simulink model "WaveletTraj"  (Simulink 10.1)
settings: Solver=FixedStepDiscrete  StartTime=0.0  StopTime=inf  FixedStep=Ts  RelTol=1e-3
PreLoadFcn:
  | load param
undefined symbols (not defined in the file or in its folder): c_maxsz, DiscIntNeverNeededParam, Dphival_fi, f, interp_gain, interp_uplim, phival_fi, Ts, tval_fi, w
libraries: simulink x36, dspsigops x24, dspindex x16, dspswit3 x12, simulink_extras x8
(part 2 of 4)

== system WaveletTraj/Wavelet Trajectory/TrajGen1/Input Latching ==
  trigger : Inport
  abort : Inport  Port=2
  mode : Inport  Port=3
  int_mode : Inport  Port=4
  Res : Inport  Port=5
  x0 : Inport  Port=6
  xf : Inport  Port=7
  T : Inport  Port=8
  c : Inport  Port=9
  Edge Detector : dspswit3/Edge Detector  SystemSampleTime=-1
      settings: SourceProductBaseCode=DS
  Edge Detector1 : dspswit3/Edge Detector  SystemSampleTime=-1
      settings: SourceProductBaseCode=DS
  Sample and Hold : Subsystem  TreatAsAtomicUnit=on  mask(Sample and Hold){trig=Rising edge, initCond=0, latchinput=off}
      mask prompts: trig "Trigger type:"; initCond "Initial condition:"; latchinput "Latch (buffer) input"
      mask help: Sample and hold the input signal. If Latch (buffer) input is selected, then this block produces the value of the input from the previous time step.
      mask init:
      | switch trig
      | case 1, s='rising';
      | case 2, s='falling';
      | case 3, s='either';
      | end
      | set_param([gcb '/Trigger'],'triggertype',s);
      | if (latchinput == 1)
      | 	set_param([gcb '/In'],'latchinput','on');
      | 	set_param([gcb '/mode'],'latchinput','on');
      | else
      | 	set_param([gcb '/In'],'latchinput','off');
      | 	set_param([gcb '/mode'],'latchinput','off');
      | end
      mask Help: eval('blocksethelp');
      mask TypeOptions trig: Rising edge | Falling edge | Either edge
      mask Display: disp('S/H')
  Sample and Hold1 : dspsigops/Sample and Hold  SystemSampleTime=-1  trig=Rising edge  initCond=0  latchinput=off
  Sample and Hold2 : Subsystem  TreatAsAtomicUnit=on  mask(Sample and Hold){trig=Rising edge, initCond=0, latchinput=off}
      mask prompts: trig "Trigger type:"; initCond "Initial condition:"; latchinput "Latch (buffer) input"
      mask help: Sample and hold the input signal. If Latch (buffer) input is selected, then this block produces the value of the input from the previous time step.
      mask init:
      | switch trig
      | case 1, s='rising';
      | case 2, s='falling';
      | case 3, s='either';
      | end
      | set_param([gcb '/Trigger'],'triggertype',s);
      | if (latchinput == 1)
      | 	set_param([gcb '/In'],'latchinput','on');
      | else
      | 	set_param([gcb '/In'],'latchinput','off');
      | end
      mask Help: eval('blocksethelp');
      mask TypeOptions trig: Rising edge | Falling edge | Either edge
      mask Display: disp('S/H')
  Sample and Hold3 : dspsigops/Sample and Hold  SystemSampleTime=-1  trig=Rising edge  initCond=0  latchinput=off
  Sample and Hold4 : Subsystem  TreatAsAtomicUnit=on  mask(Sample and Hold){trig=Rising edge, initCond=0, latchinput=off}
      mask prompts: trig "Trigger type:"; initCond "Initial condition:"; latchinput "Latch (buffer) input"
      mask help: Sample and hold the input signal. If Latch (buffer) input is selected, then this block produces the value of the input from the previous time step.
      mask init: same as WaveletTraj/Wavelet Trajectory/TrajGen1/Input Latching/Sample and Hold
      mask Help: eval('blocksethelp');
      mask TypeOptions trig: Rising edge | Falling edge | Either edge
      mask Display: disp('S/H')
  Sample and Hold5 : Subsystem  TreatAsAtomicUnit=on  mask(Sample and Hold){trig=Rising edge, initCond=0, latchinput=off}
      mask prompts: trig "Trigger type:"; initCond "Initial condition:"; latchinput "Latch (buffer) input"
      mask help: Sample and hold the input signal. If Latch (buffer) input is selected, then this block produces the value of the input from the previous time step.
      mask init:
      | switch trig
      | case 1, s='rising';
      | case 2, s='falling';
      | case 3, s='either';
      | end
      | set_param([gcb '/Trigger'],'triggertype',s);
      | if (latchinput == 1)
      | 	set_param([gcb '/mode'],'latchinput','on');
      | 	set_param([gcb '/x0'],'latchinput','on');
      | 	set_param([gcb '/xf'],'latchinput','on');
      | else
      | 	set_param([gcb '/mode'],'latchinput','off');
      | 	set_param([gcb '/x0'],'latchinput','off');
      | 	set_param([gcb '/xf'],'latchinput','off');
      | end
      mask Help: eval('blocksethelp');
      mask TypeOptions trig: Rising edge | Falling edge | Either edge
      mask Display: disp('S/H')
  Sample and Hold6 : dspsigops/Sample and Hold  SystemSampleTime=-1  trig=Rising edge  initCond=0  latchinput=off
  Saturation : Saturate  UpperLimit=2  LowerLimit=0  OutDataTypeStr=uint8  RndMeth=Nearest
  trigger_trg : Outport
  abort_trg : Outport  Port=2
  mode_lt : Outport  Port=3
  int_mode_lt : Outport  Port=4
  Res_lt : Outport  Port=5
  N_lt : Outport  Port=6
  x0_lt : Outport  Port=7
  mul_lt : Outport  Port=8
  T1 : Outport  Port=9
  c_lt : Outport  Port=10
  wires:
  Sample and Hold4/1(" ") -> c_lt/1
  Sample and Hold2/1(" ") -> T1/1
  T/1 -> Sample and Hold2/1(In)
  Sample and Hold1/1 -> x0_lt/1
  x0/1 -> Sample and Hold1/1, Sample and Hold5/2(x0)
  Sample and Hold/2(" 1") -> N_lt/1
  Res/1 -> Sample and Hold/2(In)
  Sample and Hold/1(" ") -> Res_lt/1
  Edge Detector/1 -> trigger_trg/1
  trigger/1 -> Edge Detector/1, Sample and Hold3/Trigger, Sample and Hold1/Trigger, Sample and Hold5/Trigger, Sample and Hold2/Trigger, Sample and Hold4/Trigger, Sample and Hold/Trigger, Sample and Hold6/Trigger
  mode/1 -> Saturation/1
  xf/1 -> Sample and Hold5/3(xf)
  Sample and Hold5/1(" ") -> mul_lt/1
  c/1 -> Sample and Hold4/2(In)
  abort/1 -> Edge Detector1/1
  Edge Detector1/1 -> abort_trg/1
  Sample and Hold3/1 -> mode_lt/1
  Sample and Hold6/1 -> int_mode_lt/1
  int_mode/1 -> Sample and Hold6/1
  Saturation/1 -> Sample and Hold4/1(mode), Sample and Hold5/1(mode), Sample and Hold/1(mode), Sample and Hold3/1

== system WaveletTraj/Wavelet Trajectory/TrajGen2/Compute Join Coeffs ==
  x_z1 : Inport
  tau_z1 : Inport  Port=2
  Res_z1 : Inport  Port=3
  c_z1 : Inport  Port=4
  N_z1 : Inport  Port=5
  mul_z1 : Inport  Port=6
  Res : Inport  Port=7
  c : Inport  Port=8
  N : Inport  Port=9
  mul : Inport  Port=10
  x0 : Inport  Port=11
  Trigger : TriggerPort  VariantControl=(inherit)  StatesWhenEnabling=reset
  Abs : Abs  RndMeth=Nearest  SaturateOnIntegerOverflow=on
  Constant : Constant  Value=0  OutDataTypeStr=fixdt(1,w,f)
  Derivative1 in tau : Subsystem  TreatAsAtomicUnit=on  RTWFcnName=Trajectory_Derivative
      settings: RTWFcnNameOpts=User specified
  Derivative2 in 0 : Subsystem  TreatAsAtomicUnit=on  RTWFcnName=Trajectory_Derivative
      settings: RTWFcnNameOpts=User specified
  Derivative2 in tau1 : Subsystem  TreatAsAtomicUnit=on  RTWFcnName=Trajectory_Derivative
      settings: RTWFcnNameOpts=User specified
  Find Coeffs : Subsystem  TreatAsAtomicUnit=on  RTWFcnName=Trajectory_FindCoeffs
      settings: RTWFcnNameOpts=User specified
  Gain : Gain  Gain=interp_gain  ParamDataTypeStr=fixdt(1,w,f)  RndMeth=Nearest  SaturateOnIntegerOverflow=on  OutDataTypeStr=Inherit: Same as input
  Position2 in tau1 : Subsystem  TreatAsAtomicUnit=on  RTWFcnName=Trajectory_Position
      settings: RTWFcnNameOpts=User specified
  Product{,1..3} (4 alike) : Product  OutDataTypeStr=fixdt(1,w,f)  RndMeth=Nearest  SaturateOnIntegerOverflow=on
  Saturation1 : Saturate  UpperLimit=interp_uplim  LowerLimit=0  OutDataTypeStr=fixdt(1,w,f)  RndMeth=Nearest
  Sum1 : Sum  Inputs=++|  OutDataTypeStr=fixdt(1,w,f)  RndMeth=Nearest  SaturateOnIntegerOverflow=on
  Sum2 : Sum  Inputs=|+-  OutDataTypeStr=fixdt(1,w,f)  RndMeth=Nearest  SaturateOnIntegerOverflow=on
  tau1 : Outport
  DET_OK : Outport  Port=2
  Coeffs : Outport  Port=3
  wires:
  mul/1 -> Product3/1, Product/1, Product2/1
  Position2 in tau1/1(out) -> Product/2
  Product3/1 -> [Dout2]
  Derivative2 in tau1/1(out) -> Product3/2
  Product2/1 -> Sum2/2
  Derivative2 in 0/1(out) -> Product2/2
  mul_z1/1 -> Product1/1
  Product1/1 -> [Dout1], Sum2/1
  Derivative1 in tau/1(out) -> Product1/2
  Product/1 -> Sum1/2
  Res/1 -> Position2 in tau1/1(Res), Derivative2 in tau1/1(Res), Derivative2 in 0/1(Res)
  Constant/1 -> Derivative2 in 0/2(tau)
  c/1 -> Position2 in tau1/3(c), Derivative2 in tau1/3(c), Derivative2 in 0/3(c)
  N/1 -> Position2 in tau1/4(N), Derivative2 in tau1/4(N), Derivative2 in 0/4(N)
  Sum2/1 -> Abs/1
  Abs/1 -> Gain/1
  Gain/1 -> Saturation1/1
  [tau1] -> Position2 in tau1/2(tau), Derivative2 in tau1/2(tau)
  x_z1/1 -> [out1]
  [tau1] -> Find Coeffs/1(tau1)
  [out1] -> Find Coeffs/2(out1)
  [Dout1] -> Find Coeffs/3(Dout1)
  [out2] -> Find Coeffs/4(out2)
  [Dout2] -> Find Coeffs/5(Dout2)
  Find Coeffs/2(Coeffs) -> Coeffs/1
  Saturation1/1 -> tau1/1, [tau1]
  Sum1/1 -> [out2]
  x0/1 -> Sum1/1
  c_z1/1 -> Derivative1 in tau/3(c)
  tau_z1/1 -> Derivative1 in tau/2(tau)
  Find Coeffs/1(DET_OK) -> DET_OK/1
  Res_z1/1 -> Derivative1 in tau/1(Res)
  N_z1/1 -> Derivative1 in tau/4(N)

== system WaveletTraj/Wavelet Trajectory/TrajGen2/Compute Join Output ==
  Coeffs : Inport
  tau : Inport  Port=2
  tau1 : Inport  Port=3
  x : Inport  Port=4
  Enable : EnablePort
  CalcPoly : Subsystem
  CalcRho : Subsystem
  Product : Product  OutDataTypeStr=fixdt(1,w,f)  RndMeth=Nearest  SaturateOnIntegerOverflow=on
  Product1 : Product  OutDataTypeStr=fixdt(1,w,f)  RndMeth=Nearest  SaturateOnIntegerOverflow=on
  Sum2 : Sum  Inputs=|++  OutDataTypeStr=fixdt(1,w,f)  RndMeth=Nearest  SaturateOnIntegerOverflow=on
  x_join : Outport
  wires:
  tau/1 -> CalcPoly/1(tau), CalcRho/1(tau)
  Coeffs/1 -> CalcPoly/2(Coeffs)
  tau1/1 -> CalcRho/2(tau1)
  CalcPoly/1(out_poly3) -> Product/1
  CalcRho/1(Rho1) -> Product/2
  Product/1 -> Sum2/1
  Product1/1 -> Sum2/2
  Sum2/1 -> x_join/1
  CalcRho/2(Rho2) -> Product1/1
  x/1 -> Product1/2

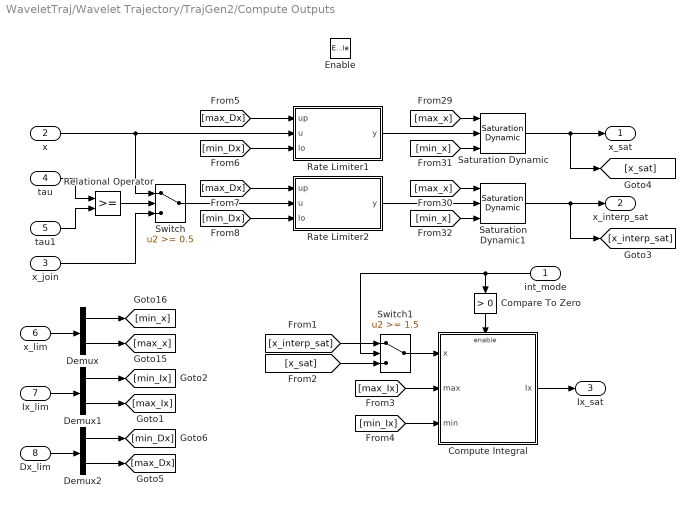
== system WaveletTraj/Wavelet Trajectory/TrajGen2/Compute Outputs ==
  int_mode : Inport
  x : Inport  Port=2
  x_join : Inport  Port=3
  tau : Inport  Port=4
  tau1 : Inport  Port=5
  x_lim : Inport  Port=6
  Ix_lim : Inport  Port=7
  Dx_lim : Inport  Port=8
  Enable : EnablePort
  Compare To Zero : simulink/Logic and Bit Operations/Compare To Zero  SystemSampleTime=-1  relop=>  LogicOutDataTypeMode=boolean  ZeroCross=off
  Compute Integral : Subsystem  TreatAsAtomicUnit=on  RTWFcnName=Trajectory_ComputeIntegral
      settings: RTWFcnNameOpts=User specified
  Demux : Demux  Outputs=2
  Demux1 : Demux  Outputs=2
  Demux2 : Demux  Outputs=2
  Rate Limiter1 : Subsystem  TreatAsAtomicUnit=on  RTWFcnName=Trajectory_RateLimiter
      settings: RTWFcnNameOpts=User specified
      mask Display:
      | disp('Rate\nLimiter');
      | port_label('input',1,'up');
      | port_label('input',2,'u');
      | port_label('input',3,'lo');
      | port_label('output',1,'y');
  Rate Limiter2 : Subsystem  TreatAsAtomicUnit=on  RTWFcnName=Trajectory_RateLimiter
      settings: RTWFcnNameOpts=User specified
      mask Display:
      | disp('Rate\nLimiter');
      | port_label('input',1,'up');
      | port_label('input',2,'u');
      | port_label('input',3,'lo');
      | port_label('output',1,'y');
  Relational Operator : RelationalOperator  OutDataTypeStr=boolean  RndMeth=Nearest
  Saturation Dynamic : simulink/Discontinuities/Saturation Dynamic  SystemSampleTime=-1  OutMin=[]  OutMax=[]  OutDataTypeStr=fixdt(1,w,f)  OutputDataTypeScalingMode=Specify via dialog  OutDataType=fixdt(1,w,f)  OutScaling=[]  RndMeth=Nearest  DoSatur=on
  Saturation Dynamic1 : simulink/Discontinuities/Saturation Dynamic  SystemSampleTime=-1  OutMin=[]  OutMax=[]  OutDataTypeStr=fixdt(1,w,f)  OutputDataTypeScalingMode=Specify via dialog  OutDataType=fixdt(1,w,f)  OutScaling=[]  RndMeth=Nearest  DoSatur=on
  Switch : Switch  Threshold=0.5  OutDataTypeStr=fixdt(1,w,f)  RndMeth=Nearest  SaturateOnIntegerOverflow=on
  Switch1 : Switch  Threshold=1.5  OutDataTypeStr=fixdt(1,w,f)  RndMeth=Nearest  SaturateOnIntegerOverflow=on
  x_sat : Outport
  x_interp_sat : Outport  Port=2
  Ix_sat : Outport  Port=3
  wires:
  [max_Dx] -> Rate Limiter2/1(up)
  [min_Dx] -> Rate Limiter2/3(lo)
  [min_Dx] -> Rate Limiter1/3(lo)
  [max_Dx] -> Rate Limiter1/1(up)
  Switch/1 -> Rate Limiter2/2(u)
  Rate Limiter2/1(y) -> Saturation Dynamic1/2
  Rate Limiter1/1(y) -> Saturation Dynamic/2
  Dx_lim/1 -> Demux2/1
  Demux2/2 -> [max_Dx]
  Demux2/1 -> [min_Dx]
  Compare To Zero/1 -> Compute Integral/Enable
  int_mode/1 -> Switch1/2, Compare To Zero/1
  Switch1/1 -> Compute Integral/1(x)
  [x_sat] -> Switch1/3
  [x_interp_sat] -> Switch1/1
  Ix_lim/1 -> Demux1/1
  x_lim/1 -> Demux/1
  Compute Integral/1(Ix) -> Ix_sat/1
  [min_Ix] -> Compute Integral/3(min)
  [max_Ix] -> Compute Integral/2(max)
  Demux1/2 -> [max_Ix]
  Demux1/1 -> [min_Ix]
  Demux/2 -> [max_x]
  Demux/1 -> [min_x]
  x_join/1 -> Switch/3
  tau1/1 -> Relational Operator/2
  Saturation Dynamic1/1 -> [x_interp_sat], x_interp_sat/1
  tau/1 -> Relational Operator/1
  Saturation Dynamic/1 -> [x_sat], x_sat/1
  Relational Operator/1 -> Switch/2
  [max_x] -> Saturation Dynamic/1
  [max_x] -> Saturation Dynamic1/1
  [min_x] -> Saturation Dynamic/3
  [min_x] -> Saturation Dynamic1/3
  x/1 -> Rate Limiter1/2(u), Switch/1

== system WaveletTraj/Wavelet Trajectory/TrajGen2/Compute Position ==
  Res : Inport  PortDimensions=1
  tau : Inport  Port=2  PortDimensions=1
  c : Inport  Port=3  PortDimensions=c_maxsz
  N : Inport  Port=4  PortDimensions=1
  mul : Inport  Port=5  PortDimensions=1
  x0 : Inport  Port=6  PortDimensions=1
  Enable : EnablePort
  Position : Subsystem  TreatAsAtomicUnit=on  RTWFcnName=Trajectory_Position
      settings: RTWFcnNameOpts=User specified
  Product : Product  OutDataTypeStr=fixdt(1,w,f)  RndMeth=Nearest  SaturateOnIntegerOverflow=on
  Sum1 : Sum  Inputs=|++  OutDataTypeStr=fixdt(1,w,f)  RndMeth=Nearest  SaturateOnIntegerOverflow=on
  out : Outport  PortDimensions=1
  wires:
  mul/1 -> Product/2
  Product/1 -> Sum1/1
  Position/1(out) -> Product/1
  Res/1 -> Position/1(Res)
  tau/1 -> Position/2(tau)
  c/1 -> Position/3(c)
  N/1 -> Position/4(N)
  Sum1/1 -> out/1
  x0/1 -> Sum1/2

== system WaveletTraj/Wavelet Trajectory/TrajGen2/Input Latching ==
  trigger : Inport
  abort : Inport  Port=2
  mode : Inport  Port=3
  int_mode : Inport  Port=4
  Res : Inport  Port=5
  x0 : Inport  Port=6
  xf : Inport  Port=7
  T : Inport  Port=8
  c : Inport  Port=9
  Edge Detector : dspswit3/Edge Detector  SystemSampleTime=-1
      settings: SourceProductBaseCode=DS
  Edge Detector1 : dspswit3/Edge Detector  SystemSampleTime=-1
      settings: SourceProductBaseCode=DS
  Sample and Hold : Subsystem  TreatAsAtomicUnit=on  mask(Sample and Hold){trig=Rising edge, initCond=0, latchinput=off}
      mask prompts: trig "Trigger type:"; initCond "Initial condition:"; latchinput "Latch (buffer) input"
      mask help: Sample and hold the input signal. If Latch (buffer) input is selected, then this block produces the value of the input from the previous time step.
      mask init: same as WaveletTraj/Wavelet Trajectory/TrajGen1/Input Latching/Sample and Hold
      mask Help: eval('blocksethelp');
      mask TypeOptions trig: Rising edge | Falling edge | Either edge
      mask Display: disp('S/H')
  Sample and Hold1 : dspsigops/Sample and Hold  SystemSampleTime=-1  trig=Rising edge  initCond=0  latchinput=off
  Sample and Hold2 : Subsystem  TreatAsAtomicUnit=on  mask(Sample and Hold){trig=Rising edge, initCond=0, latchinput=off}
      mask prompts: trig "Trigger type:"; initCond "Initial condition:"; latchinput "Latch (buffer) input"
      mask help: Sample and hold the input signal. If Latch (buffer) input is selected, then this block produces the value of the input from the previous time step.
      mask init: same as WaveletTraj/Wavelet Trajectory/TrajGen1/Input Latching/Sample and Hold2
      mask Help: eval('blocksethelp');
      mask TypeOptions trig: Rising edge | Falling edge | Either edge
      mask Display: disp('S/H')
  Sample and Hold3 : dspsigops/Sample and Hold  SystemSampleTime=-1  trig=Rising edge  initCond=0  latchinput=off
  Sample and Hold4 : Subsystem  TreatAsAtomicUnit=on  mask(Sample and Hold){trig=Rising edge, initCond=0, latchinput=off}
      mask prompts: trig "Trigger type:"; initCond "Initial condition:"; latchinput "Latch (buffer) input"
      mask help: Sample and hold the input signal. If Latch (buffer) input is selected, then this block produces the value of the input from the previous time step.
      mask init: same as WaveletTraj/Wavelet Trajectory/TrajGen1/Input Latching/Sample and Hold
      mask Help: eval('blocksethelp');
      mask TypeOptions trig: Rising edge | Falling edge | Either edge
      mask Display: disp('S/H')
  Sample and Hold5 : Subsystem  TreatAsAtomicUnit=on  mask(Sample and Hold){trig=Rising edge, initCond=0, latchinput=off}
      mask prompts: trig "Trigger type:"; initCond "Initial condition:"; latchinput "Latch (buffer) input"
      mask help: Sample and hold the input signal. If Latch (buffer) input is selected, then this block produces the value of the input from the previous time step.
      mask init: same as WaveletTraj/Wavelet Trajectory/TrajGen1/Input Latching/Sample and Hold5
      mask Help: eval('blocksethelp');
      mask TypeOptions trig: Rising edge | Falling edge | Either edge
      mask Display: disp('S/H')
  Sample and Hold6 : dspsigops/Sample and Hold  SystemSampleTime=-1  trig=Rising edge  initCond=0  latchinput=off
  Saturation : Saturate  UpperLimit=2  LowerLimit=0  OutDataTypeStr=uint8  RndMeth=Nearest
  trigger_trg : Outport
  abort_trg : Outport  Port=2
  mode_lt : Outport  Port=3
  int_mode_lt : Outport  Port=4
  Res_lt : Outport  Port=5
  N_lt : Outport  Port=6
  x0_lt : Outport  Port=7
  mul_lt : Outport  Port=8
  T1 : Outport  Port=9
  c_lt : Outport  Port=10
  wires:
  Saturation/1 -> Sample and Hold3/1, Sample and Hold/1(mode), Sample and Hold5/1(mode), Sample and Hold4/1(mode)
  int_mode/1 -> Sample and Hold6/1
  Sample and Hold6/1 -> int_mode_lt/1
  Sample and Hold3/1 -> mode_lt/1
  Edge Detector1/1 -> abort_trg/1
  abort/1 -> Edge Detector1/1
  c/1 -> Sample and Hold4/2(In)
  Sample and Hold5/1(" ") -> mul_lt/1
  xf/1 -> Sample and Hold5/3(xf)
  mode/1 -> Saturation/1
  trigger/1 -> Sample and Hold6/Trigger, Sample and Hold/Trigger, Sample and Hold4/Trigger, Sample and Hold2/Trigger, Sample and Hold5/Trigger, Sample and Hold1/Trigger, Sample and Hold3/Trigger, Edge Detector/1
  Edge Detector/1 -> trigger_trg/1
  Sample and Hold/1(" ") -> Res_lt/1
  Res/1 -> Sample and Hold/2(In)
  Sample and Hold/2(" 1") -> N_lt/1
  x0/1 -> Sample and Hold5/2(x0), Sample and Hold1/1
  Sample and Hold1/1 -> x0_lt/1
  T/1 -> Sample and Hold2/1(In)
  Sample and Hold2/1(" ") -> T1/1
  Sample and Hold4/1(" ") -> c_lt/1

== system WaveletTraj/Wavelet Trajectory/TrajGen3/Compute Join Coeffs ==
  x_z1 : Inport
  tau_z1 : Inport  Port=2
  Res_z1 : Inport  Port=3
  c_z1 : Inport  Port=4
  N_z1 : Inport  Port=5
  mul_z1 : Inport  Port=6
  Res : Inport  Port=7
  c : Inport  Port=8
  N : Inport  Port=9
  mul : Inport  Port=10
  x0 : Inport  Port=11
  Trigger : TriggerPort  VariantControl=(inherit)  StatesWhenEnabling=reset
  Abs : Abs  RndMeth=Nearest  SaturateOnIntegerOverflow=on
  Constant : Constant  Value=0  OutDataTypeStr=fixdt(1,w,f)
  Derivative1 in tau : Subsystem  TreatAsAtomicUnit=on  RTWFcnName=Trajectory_Derivative
      settings: RTWFcnNameOpts=User specified
  Derivative2 in 0 : Subsystem  TreatAsAtomicUnit=on  RTWFcnName=Trajectory_Derivative
      settings: RTWFcnNameOpts=User specified
  Derivative2 in tau1 : Subsystem  TreatAsAtomicUnit=on  RTWFcnName=Trajectory_Derivative
      settings: RTWFcnNameOpts=User specified
  Find Coeffs : Subsystem  TreatAsAtomicUnit=on  RTWFcnName=Trajectory_FindCoeffs
      settings: RTWFcnNameOpts=User specified
  Gain : Gain  Gain=interp_gain  ParamDataTypeStr=fixdt(1,w,f)  RndMeth=Nearest  SaturateOnIntegerOverflow=on  OutDataTypeStr=Inherit: Same as input
  Position2 in tau1 : Subsystem  TreatAsAtomicUnit=on  RTWFcnName=Trajectory_Position
      settings: RTWFcnNameOpts=User specified
  Product{,1..3} (4 alike) : Product  OutDataTypeStr=fixdt(1,w,f)  RndMeth=Nearest  SaturateOnIntegerOverflow=on
  Saturation1 : Saturate  UpperLimit=interp_uplim  LowerLimit=0  OutDataTypeStr=fixdt(1,w,f)  RndMeth=Nearest
  Sum1 : Sum  Inputs=++|  OutDataTypeStr=fixdt(1,w,f)  RndMeth=Nearest  SaturateOnIntegerOverflow=on
  Sum2 : Sum  Inputs=|+-  OutDataTypeStr=fixdt(1,w,f)  RndMeth=Nearest  SaturateOnIntegerOverflow=on
  tau1 : Outport
  DET_OK : Outport  Port=2
  Coeffs : Outport  Port=3
  wires:
  N_z1/1 -> Derivative1 in tau/4(N)
  Res_z1/1 -> Derivative1 in tau/1(Res)
  Find Coeffs/1(DET_OK) -> DET_OK/1
  tau_z1/1 -> Derivative1 in tau/2(tau)
  c_z1/1 -> Derivative1 in tau/3(c)
  x0/1 -> Sum1/1
  Sum1/1 -> [out2]
  Saturation1/1 -> [tau1], tau1/1
  Find Coeffs/2(Coeffs) -> Coeffs/1
  [Dout2] -> Find Coeffs/5(Dout2)
  [out2] -> Find Coeffs/4(out2)
  [Dout1] -> Find Coeffs/3(Dout1)
  [out1] -> Find Coeffs/2(out1)
  [tau1] -> Find Coeffs/1(tau1)
  x_z1/1 -> [out1]
  [tau1] -> Derivative2 in tau1/2(tau), Position2 in tau1/2(tau)
  Gain/1 -> Saturation1/1
  Abs/1 -> Gain/1
  Sum2/1 -> Abs/1
  N/1 -> Derivative2 in 0/4(N), Derivative2 in tau1/4(N), Position2 in tau1/4(N)
  c/1 -> Derivative2 in 0/3(c), Derivative2 in tau1/3(c), Position2 in tau1/3(c)
  Constant/1 -> Derivative2 in 0/2(tau)
  Res/1 -> Derivative2 in 0/1(Res), Derivative2 in tau1/1(Res), Position2 in tau1/1(Res)
  Product/1 -> Sum1/2
  Derivative1 in tau/1(out) -> Product1/2
  Product1/1 -> Sum2/1, [Dout1]
  mul_z1/1 -> Product1/1
  Derivative2 in 0/1(out) -> Product2/2
  Product2/1 -> Sum2/2
  Derivative2 in tau1/1(out) -> Product3/2
  Product3/1 -> [Dout2]
  Position2 in tau1/1(out) -> Product/2
  mul/1 -> Product2/1, Product/1, Product3/1

== system WaveletTraj/Wavelet Trajectory/TrajGen3/Compute Join Output ==
  Coeffs : Inport
  tau : Inport  Port=2
  tau1 : Inport  Port=3
  x : Inport  Port=4
  Enable : EnablePort
  CalcPoly : Subsystem
  CalcRho : Subsystem
  Product : Product  OutDataTypeStr=fixdt(1,w,f)  RndMeth=Nearest  SaturateOnIntegerOverflow=on
  Product1 : Product  OutDataTypeStr=fixdt(1,w,f)  RndMeth=Nearest  SaturateOnIntegerOverflow=on
  Sum2 : Sum  Inputs=|++  OutDataTypeStr=fixdt(1,w,f)  RndMeth=Nearest  SaturateOnIntegerOverflow=on
  x_join : Outport
  wires:
  x/1 -> Product1/2
  CalcRho/2(Rho2) -> Product1/1
  Sum2/1 -> x_join/1
  Product1/1 -> Sum2/2
  Product/1 -> Sum2/1
  CalcRho/1(Rho1) -> Product/2
  CalcPoly/1(out_poly3) -> Product/1
  tau1/1 -> CalcRho/2(tau1)
  Coeffs/1 -> CalcPoly/2(Coeffs)
  tau/1 -> CalcRho/1(tau), CalcPoly/1(tau)

== system WaveletTraj/Wavelet Trajectory/TrajGen3/Compute Outputs ==
  int_mode : Inport
  x : Inport  Port=2
  x_join : Inport  Port=3
  tau : Inport  Port=4
  tau1 : Inport  Port=5
  x_lim : Inport  Port=6
  Ix_lim : Inport  Port=7
  Dx_lim : Inport  Port=8
  Enable : EnablePort
  Compare To Zero : simulink/Logic and Bit Operations/Compare To Zero  SystemSampleTime=-1  relop=>  LogicOutDataTypeMode=boolean  ZeroCross=off
  Compute Integral : Subsystem  TreatAsAtomicUnit=on  RTWFcnName=Trajectory_ComputeIntegral
      settings: RTWFcnNameOpts=User specified
  Demux : Demux  Outputs=2
  Demux1 : Demux  Outputs=2
  Demux2 : Demux  Outputs=2
  Rate Limiter1 : Subsystem  TreatAsAtomicUnit=on  RTWFcnName=Trajectory_RateLimiter
      settings: RTWFcnNameOpts=User specified
      mask Display:
      | disp('Rate\nLimiter');
      | port_label('input',1,'up');
      | port_label('input',2,'u');
      | port_label('input',3,'lo');
      | port_label('output',1,'y');
  Rate Limiter2 : Subsystem  TreatAsAtomicUnit=on  RTWFcnName=Trajectory_RateLimiter
      settings: RTWFcnNameOpts=User specified
      mask Display:
      | disp('Rate\nLimiter');
      | port_label('input',1,'up');
      | port_label('input',2,'u');
      | port_label('input',3,'lo');
      | port_label('output',1,'y');
  Relational Operator : RelationalOperator  OutDataTypeStr=boolean  RndMeth=Nearest
  Saturation Dynamic : simulink/Discontinuities/Saturation Dynamic  SystemSampleTime=-1  OutMin=[]  OutMax=[]  OutDataTypeStr=fixdt(1,w,f)  OutputDataTypeScalingMode=Specify via dialog  OutDataType=fixdt(1,w,f)  OutScaling=[]  RndMeth=Nearest  DoSatur=on
  Saturation Dynamic1 : simulink/Discontinuities/Saturation Dynamic  SystemSampleTime=-1  OutMin=[]  OutMax=[]  OutDataTypeStr=fixdt(1,w,f)  OutputDataTypeScalingMode=Specify via dialog  OutDataType=fixdt(1,w,f)  OutScaling=[]  RndMeth=Nearest  DoSatur=on
  Switch : Switch  Threshold=0.5  OutDataTypeStr=fixdt(1,w,f)  RndMeth=Nearest  SaturateOnIntegerOverflow=on
  Switch1 : Switch  Threshold=1.5  OutDataTypeStr=fixdt(1,w,f)  RndMeth=Nearest  SaturateOnIntegerOverflow=on
  x_sat : Outport
  x_interp_sat : Outport  Port=2
  Ix_sat : Outport  Port=3
  wires:
  x/1 -> Switch/1, Rate Limiter1/2(u)
  [min_x] -> Saturation Dynamic1/3
  [min_x] -> Saturation Dynamic/3
  [max_x] -> Saturation Dynamic1/1
  [max_x] -> Saturation Dynamic/1
  Relational Operator/1 -> Switch/2
  Saturation Dynamic/1 -> x_sat/1, [x_sat]
  tau/1 -> Relational Operator/1
  Saturation Dynamic1/1 -> x_interp_sat/1, [x_interp_sat]
  tau1/1 -> Relational Operator/2
  x_join/1 -> Switch/3
  Demux/1 -> [min_x]
  Demux/2 -> [max_x]
  Demux1/1 -> [min_Ix]
  Demux1/2 -> [max_Ix]
  [max_Ix] -> Compute Integral/2(max)
  [min_Ix] -> Compute Integral/3(min)
  Compute Integral/1(Ix) -> Ix_sat/1
  x_lim/1 -> Demux/1
  Ix_lim/1 -> Demux1/1
  [x_interp_sat] -> Switch1/1
  [x_sat] -> Switch1/3
  Switch1/1 -> Compute Integral/1(x)
  int_mode/1 -> Compare To Zero/1, Switch1/2
  Compare To Zero/1 -> Compute Integral/Enable
  Demux2/1 -> [min_Dx]
  Demux2/2 -> [max_Dx]
  Dx_lim/1 -> Demux2/1
  Rate Limiter1/1(y) -> Saturation Dynamic/2
  Rate Limiter2/1(y) -> Saturation Dynamic1/2
  Switch/1 -> Rate Limiter2/2(u)
  [max_Dx] -> Rate Limiter1/1(up)
  [min_Dx] -> Rate Limiter1/3(lo)
  [min_Dx] -> Rate Limiter2/3(lo)
  [max_Dx] -> Rate Limiter2/1(up)

== system WaveletTraj/Wavelet Trajectory/TrajGen3/Compute Position ==
  Res : Inport  PortDimensions=1
  tau : Inport  Port=2  PortDimensions=1
  c : Inport  Port=3  PortDimensions=c_maxsz
  N : Inport  Port=4  PortDimensions=1
  mul : Inport  Port=5  PortDimensions=1
  x0 : Inport  Port=6  PortDimensions=1
  Enable : EnablePort
  Position : Subsystem  TreatAsAtomicUnit=on  RTWFcnName=Trajectory_Position
      settings: RTWFcnNameOpts=User specified
  Product : Product  OutDataTypeStr=fixdt(1,w,f)  RndMeth=Nearest  SaturateOnIntegerOverflow=on
  Sum1 : Sum  Inputs=|++  OutDataTypeStr=fixdt(1,w,f)  RndMeth=Nearest  SaturateOnIntegerOverflow=on
  out : Outport  PortDimensions=1
  wires:
  x0/1 -> Sum1/2
  Sum1/1 -> out/1
  N/1 -> Position/4(N)
  c/1 -> Position/3(c)
  tau/1 -> Position/2(tau)
  Res/1 -> Position/1(Res)
  Position/1(out) -> Product/1
  Product/1 -> Sum1/1
  mul/1 -> Product/2

== system WaveletTraj/Wavelet Trajectory/TrajGen3/Input Latching ==
  trigger : Inport
  abort : Inport  Port=2
  mode : Inport  Port=3
  int_mode : Inport  Port=4
  Res : Inport  Port=5
  x0 : Inport  Port=6
  xf : Inport  Port=7
  T : Inport  Port=8
  c : Inport  Port=9
  Edge Detector : dspswit3/Edge Detector  SystemSampleTime=-1
      settings: SourceProductBaseCode=DS
  Edge Detector1 : dspswit3/Edge Detector  SystemSampleTime=-1
      settings: SourceProductBaseCode=DS
  Sample and Hold : Subsystem  TreatAsAtomicUnit=on  mask(Sample and Hold){trig=Rising edge, initCond=0, latchinput=off}
      mask prompts: trig "Trigger type:"; initCond "Initial condition:"; latchinput "Latch (buffer) input"
      mask help: Sample and hold the input signal. If Latch (buffer) input is selected, then this block produces the value of the input from the previous time step.
      mask init: same as WaveletTraj/Wavelet Trajectory/TrajGen1/Input Latching/Sample and Hold
      mask Help: eval('blocksethelp');
      mask TypeOptions trig: Rising edge | Falling edge | Either edge
      mask Display: disp('S/H')
  Sample and Hold1 : dspsigops/Sample and Hold  SystemSampleTime=-1  trig=Rising edge  initCond=0  latchinput=off
  Sample and Hold2 : Subsystem  TreatAsAtomicUnit=on  mask(Sample and Hold){trig=Rising edge, initCond=0, latchinput=off}
      mask prompts: trig "Trigger type:"; initCond "Initial condition:"; latchinput "Latch (buffer) input"
      mask help: Sample and hold the input signal. If Latch (buffer) input is selected, then this block produces the value of the input from the previous time step.
      mask init: same as WaveletTraj/Wavelet Trajectory/TrajGen1/Input Latching/Sample and Hold2
      mask Help: eval('blocksethelp');
      mask TypeOptions trig: Rising edge | Falling edge | Either edge
      mask Display: disp('S/H')
  Sample and Hold3 : dspsigops/Sample and Hold  SystemSampleTime=-1  trig=Rising edge  initCond=0  latchinput=off
  Sample and Hold4 : Subsystem  TreatAsAtomicUnit=on  mask(Sample and Hold){trig=Rising edge, initCond=0, latchinput=off}
      mask prompts: trig "Trigger type:"; initCond "Initial condition:"; latchinput "Latch (buffer) input"
      mask help: Sample and hold the input signal. If Latch (buffer) input is selected, then this block produces the value of the input from the previous time step.
      mask init: same as WaveletTraj/Wavelet Trajectory/TrajGen1/Input Latching/Sample and Hold
      mask Help: eval('blocksethelp');
      mask TypeOptions trig: Rising edge | Falling edge | Either edge
      mask Display: disp('S/H')
  Sample and Hold5 : Subsystem  TreatAsAtomicUnit=on  mask(Sample and Hold){trig=Rising edge, initCond=0, latchinput=off}
      mask prompts: trig "Trigger type:"; initCond "Initial condition:"; latchinput "Latch (buffer) input"
      mask help: Sample and hold the input signal. If Latch (buffer) input is selected, then this block produces the value of the input from the previous time step.
      mask init: same as WaveletTraj/Wavelet Trajectory/TrajGen1/Input Latching/Sample and Hold5
      mask Help: eval('blocksethelp');
      mask TypeOptions trig: Rising edge | Falling edge | Either edge
      mask Display: disp('S/H')
  Sample and Hold6 : dspsigops/Sample and Hold  SystemSampleTime=-1  trig=Rising edge  initCond=0  latchinput=off
  Saturation : Saturate  UpperLimit=2  LowerLimit=0  OutDataTypeStr=uint8  RndMeth=Nearest
  trigger_trg : Outport
  abort_trg : Outport  Port=2
  mode_lt : Outport  Port=3
  int_mode_lt : Outport  Port=4
  Res_lt : Outport  Port=5
  N_lt : Outport  Port=6
  x0_lt : Outport  Port=7
  mul_lt : Outport  Port=8
  T1 : Outport  Port=9
  c_lt : Outport  Port=10
  wires:
  Sample and Hold4/1(" ") -> c_lt/1
  Sample and Hold2/1(" ") -> T1/1
  T/1 -> Sample and Hold2/1(In)
  Sample and Hold1/1 -> x0_lt/1
  x0/1 -> Sample and Hold1/1, Sample and Hold5/2(x0)
  Sample and Hold/2(" 1") -> N_lt/1
  Res/1 -> Sample and Hold/2(In)
  Sample and Hold/1(" ") -> Res_lt/1
  Edge Detector/1 -> trigger_trg/1
  trigger/1 -> Edge Detector/1, Sample and Hold3/Trigger, Sample and Hold1/Trigger, Sample and Hold5/Trigger, Sample and Hold2/Trigger, Sample and Hold4/Trigger, Sample and Hold/Trigger, Sample and Hold6/Trigger
  mode/1 -> Saturation/1
  xf/1 -> Sample and Hold5/3(xf)
  Sample and Hold5/1(" ") -> mul_lt/1
  c/1 -> Sample and Hold4/2(In)
  abort/1 -> Edge Detector1/1
  Edge Detector1/1 -> abort_trg/1
  Sample and Hold3/1 -> mode_lt/1
  Sample and Hold6/1 -> int_mode_lt/1
  int_mode/1 -> Sample and Hold6/1
  Saturation/1 -> Sample and Hold4/1(mode), Sample and Hold5/1(mode), Sample and Hold/1(mode), Sample and Hold3/1

== system WaveletTraj/Wavelet Trajectory/TrajGen4/Compute Join Coeffs ==
  x_z1 : Inport
  tau_z1 : Inport  Port=2
  Res_z1 : Inport  Port=3
  c_z1 : Inport  Port=4
  N_z1 : Inport  Port=5
  mul_z1 : Inport  Port=6
  Res : Inport  Port=7
  c : Inport  Port=8
  N : Inport  Port=9
  mul : Inport  Port=10
  x0 : Inport  Port=11
  Trigger : TriggerPort  VariantControl=(inherit)  StatesWhenEnabling=reset
  Abs : Abs  RndMeth=Nearest  SaturateOnIntegerOverflow=on
  Constant : Constant  Value=0  OutDataTypeStr=fixdt(1,w,f)
  Derivative1 in tau : Subsystem  TreatAsAtomicUnit=on  RTWFcnName=Trajectory_Derivative
      settings: RTWFcnNameOpts=User specified
  Derivative2 in 0 : Subsystem  TreatAsAtomicUnit=on  RTWFcnName=Trajectory_Derivative
      settings: RTWFcnNameOpts=User specified
  Derivative2 in tau1 : Subsystem  TreatAsAtomicUnit=on  RTWFcnName=Trajectory_Derivative
      settings: RTWFcnNameOpts=User specified
  Find Coeffs : Subsystem  TreatAsAtomicUnit=on  RTWFcnName=Trajectory_FindCoeffs
      settings: RTWFcnNameOpts=User specified
  Gain : Gain  Gain=interp_gain  ParamDataTypeStr=fixdt(1,w,f)  RndMeth=Nearest  SaturateOnIntegerOverflow=on  OutDataTypeStr=Inherit: Same as input
  Position2 in tau1 : Subsystem  TreatAsAtomicUnit=on  RTWFcnName=Trajectory_Position
      settings: RTWFcnNameOpts=User specified
  Product{,1..3} (4 alike) : Product  OutDataTypeStr=fixdt(1,w,f)  RndMeth=Nearest  SaturateOnIntegerOverflow=on
  Saturation1 : Saturate  UpperLimit=interp_uplim  LowerLimit=0  OutDataTypeStr=fixdt(1,w,f)  RndMeth=Nearest
  Sum1 : Sum  Inputs=++|  OutDataTypeStr=fixdt(1,w,f)  RndMeth=Nearest  SaturateOnIntegerOverflow=on
  Sum2 : Sum  Inputs=|+-  OutDataTypeStr=fixdt(1,w,f)  RndMeth=Nearest  SaturateOnIntegerOverflow=on
  tau1 : Outport
  DET_OK : Outport  Port=2
  Coeffs : Outport  Port=3
  wires:
  mul/1 -> Product3/1, Product/1, Product2/1
  Position2 in tau1/1(out) -> Product/2
  Product3/1 -> [Dout2]
  Derivative2 in tau1/1(out) -> Product3/2
  Product2/1 -> Sum2/2
  Derivative2 in 0/1(out) -> Product2/2
  mul_z1/1 -> Product1/1
  Product1/1 -> [Dout1], Sum2/1
  Derivative1 in tau/1(out) -> Product1/2
  Product/1 -> Sum1/2
  Res/1 -> Position2 in tau1/1(Res), Derivative2 in tau1/1(Res), Derivative2 in 0/1(Res)
  Constant/1 -> Derivative2 in 0/2(tau)
  c/1 -> Position2 in tau1/3(c), Derivative2 in tau1/3(c), Derivative2 in 0/3(c)
  N/1 -> Position2 in tau1/4(N), Derivative2 in tau1/4(N), Derivative2 in 0/4(N)
  Sum2/1 -> Abs/1
  Abs/1 -> Gain/1
  Gain/1 -> Saturation1/1
  [tau1] -> Position2 in tau1/2(tau), Derivative2 in tau1/2(tau)
  x_z1/1 -> [out1]
  [tau1] -> Find Coeffs/1(tau1)
  [out1] -> Find Coeffs/2(out1)
  [Dout1] -> Find Coeffs/3(Dout1)
  [out2] -> Find Coeffs/4(out2)
  [Dout2] -> Find Coeffs/5(Dout2)
  Find Coeffs/2(Coeffs) -> Coeffs/1
  Saturation1/1 -> tau1/1, [tau1]
  Sum1/1 -> [out2]
  x0/1 -> Sum1/1
  c_z1/1 -> Derivative1 in tau/3(c)
  tau_z1/1 -> Derivative1 in tau/2(tau)
  Find Coeffs/1(DET_OK) -> DET_OK/1
  Res_z1/1 -> Derivative1 in tau/1(Res)
  N_z1/1 -> Derivative1 in tau/4(N)

== system WaveletTraj/Wavelet Trajectory/TrajGen4/Compute Join Output ==
  Coeffs : Inport
  tau : Inport  Port=2
  tau1 : Inport  Port=3
  x : Inport  Port=4
  Enable : EnablePort
  CalcPoly : Subsystem
  CalcRho : Subsystem
  Product : Product  OutDataTypeStr=fixdt(1,w,f)  RndMeth=Nearest  SaturateOnIntegerOverflow=on
  Product1 : Product  OutDataTypeStr=fixdt(1,w,f)  RndMeth=Nearest  SaturateOnIntegerOverflow=on
  Sum2 : Sum  Inputs=|++  OutDataTypeStr=fixdt(1,w,f)  RndMeth=Nearest  SaturateOnIntegerOverflow=on
  x_join : Outport
  wires:
  tau/1 -> CalcPoly/1(tau), CalcRho/1(tau)
  Coeffs/1 -> CalcPoly/2(Coeffs)
  tau1/1 -> CalcRho/2(tau1)
  CalcPoly/1(out_poly3) -> Product/1
  CalcRho/1(Rho1) -> Product/2
  Product/1 -> Sum2/1
  Product1/1 -> Sum2/2
  Sum2/1 -> x_join/1
  CalcRho/2(Rho2) -> Product1/1
  x/1 -> Product1/2

== system WaveletTraj/Wavelet Trajectory/TrajGen4/Compute Outputs ==
  int_mode : Inport
  x : Inport  Port=2
  x_join : Inport  Port=3
  tau : Inport  Port=4
  tau1 : Inport  Port=5
  x_lim : Inport  Port=6
  Ix_lim : Inport  Port=7
  Dx_lim : Inport  Port=8
  Enable : EnablePort
  Compare To Zero : simulink/Logic and Bit Operations/Compare To Zero  SystemSampleTime=-1  relop=>  LogicOutDataTypeMode=boolean  ZeroCross=off
  Compute Integral : Subsystem  TreatAsAtomicUnit=on  RTWFcnName=Trajectory_ComputeIntegral
      settings: RTWFcnNameOpts=User specified
  Demux : Demux  Outputs=2
  Demux1 : Demux  Outputs=2
  Demux2 : Demux  Outputs=2
  Rate Limiter1 : Subsystem  TreatAsAtomicUnit=on  RTWFcnName=Trajectory_RateLimiter
      settings: RTWFcnNameOpts=User specified
      mask Display:
      | disp('Rate\nLimiter');
      | port_label('input',1,'up');
      | port_label('input',2,'u');
      | port_label('input',3,'lo');
      | port_label('output',1,'y');
  Rate Limiter2 : Subsystem  TreatAsAtomicUnit=on  RTWFcnName=Trajectory_RateLimiter
      settings: RTWFcnNameOpts=User specified
      mask Display:
      | disp('Rate\nLimiter');
      | port_label('input',1,'up');
      | port_label('input',2,'u');
      | port_label('input',3,'lo');
      | port_label('output',1,'y');
  Relational Operator : RelationalOperator  OutDataTypeStr=boolean  RndMeth=Nearest
  Saturation Dynamic : simulink/Discontinuities/Saturation Dynamic  SystemSampleTime=-1  OutMin=[]  OutMax=[]  OutDataTypeStr=fixdt(1,w,f)  OutputDataTypeScalingMode=Specify via dialog  OutDataType=fixdt(1,w,f)  OutScaling=[]  RndMeth=Nearest  DoSatur=on
  Saturation Dynamic1 : simulink/Discontinuities/Saturation Dynamic  SystemSampleTime=-1  OutMin=[]  OutMax=[]  OutDataTypeStr=fixdt(1,w,f)  OutputDataTypeScalingMode=Specify via dialog  OutDataType=fixdt(1,w,f)  OutScaling=[]  RndMeth=Nearest  DoSatur=on
  Switch : Switch  Threshold=0.5  OutDataTypeStr=fixdt(1,w,f)  RndMeth=Nearest  SaturateOnIntegerOverflow=on
  Switch1 : Switch  Threshold=1.5  OutDataTypeStr=fixdt(1,w,f)  RndMeth=Nearest  SaturateOnIntegerOverflow=on
  x_sat : Outport
  x_interp_sat : Outport  Port=2
  Ix_sat : Outport  Port=3
  wires:
  [max_Dx] -> Rate Limiter2/1(up)
  [min_Dx] -> Rate Limiter2/3(lo)
  [min_Dx] -> Rate Limiter1/3(lo)
  [max_Dx] -> Rate Limiter1/1(up)
  Switch/1 -> Rate Limiter2/2(u)
  Rate Limiter2/1(y) -> Saturation Dynamic1/2
  Rate Limiter1/1(y) -> Saturation Dynamic/2
  Dx_lim/1 -> Demux2/1
  Demux2/2 -> [max_Dx]
  Demux2/1 -> [min_Dx]
  Compare To Zero/1 -> Compute Integral/Enable
  int_mode/1 -> Switch1/2, Compare To Zero/1
  Switch1/1 -> Compute Integral/1(x)
  [x_sat] -> Switch1/3
  [x_interp_sat] -> Switch1/1
  Ix_lim/1 -> Demux1/1
  x_lim/1 -> Demux/1
  Compute Integral/1(Ix) -> Ix_sat/1
  [min_Ix] -> Compute Integral/3(min)
  [max_Ix] -> Compute Integral/2(max)
  Demux1/2 -> [max_Ix]
  Demux1/1 -> [min_Ix]
  Demux/2 -> [max_x]
  Demux/1 -> [min_x]
  x_join/1 -> Switch/3
  tau1/1 -> Relational Operator/2
  Saturation Dynamic1/1 -> [x_interp_sat], x_interp_sat/1
  tau/1 -> Relational Operator/1
  Saturation Dynamic/1 -> [x_sat], x_sat/1
  Relational Operator/1 -> Switch/2
  [max_x] -> Saturation Dynamic/1
  [max_x] -> Saturation Dynamic1/1
  [min_x] -> Saturation Dynamic/3
  [min_x] -> Saturation Dynamic1/3
  x/1 -> Rate Limiter1/2(u), Switch/1

== system WaveletTraj/Wavelet Trajectory/TrajGen4/Compute Position ==
  Res : Inport  PortDimensions=1
  tau : Inport  Port=2  PortDimensions=1
  c : Inport  Port=3  PortDimensions=c_maxsz
  N : Inport  Port=4  PortDimensions=1
  mul : Inport  Port=5  PortDimensions=1
  x0 : Inport  Port=6  PortDimensions=1
  Enable : EnablePort
  Position : Subsystem  TreatAsAtomicUnit=on  RTWFcnName=Trajectory_Position
      settings: RTWFcnNameOpts=User specified
  Product : Product  OutDataTypeStr=fixdt(1,w,f)  RndMeth=Nearest  SaturateOnIntegerOverflow=on
  Sum1 : Sum  Inputs=|++  OutDataTypeStr=fixdt(1,w,f)  RndMeth=Nearest  SaturateOnIntegerOverflow=on
  out : Outport  PortDimensions=1
  wires:
  mul/1 -> Product/2
  Product/1 -> Sum1/1
  Position/1(out) -> Product/1
  Res/1 -> Position/1(Res)
  tau/1 -> Position/2(tau)
  c/1 -> Position/3(c)
  N/1 -> Position/4(N)
  Sum1/1 -> out/1
  x0/1 -> Sum1/2

== system WaveletTraj/Wavelet Trajectory/TrajGen4/Input Latching ==
  trigger : Inport
  abort : Inport  Port=2
  mode : Inport  Port=3
  int_mode : Inport  Port=4
  Res : Inport  Port=5
  x0 : Inport  Port=6
  xf : Inport  Port=7
  T : Inport  Port=8
  c : Inport  Port=9
  Edge Detector : dspswit3/Edge Detector  SystemSampleTime=-1
      settings: SourceProductBaseCode=DS
  Edge Detector1 : dspswit3/Edge Detector  SystemSampleTime=-1
      settings: SourceProductBaseCode=DS
  Sample and Hold : Subsystem  TreatAsAtomicUnit=on  mask(Sample and Hold){trig=Rising edge, initCond=0, latchinput=off}
      mask prompts: trig "Trigger type:"; initCond "Initial condition:"; latchinput "Latch (buffer) input"
      mask help: Sample and hold the input signal. If Latch (buffer) input is selected, then this block produces the value of the input from the previous time step.
      mask init: same as WaveletTraj/Wavelet Trajectory/TrajGen1/Input Latching/Sample and Hold
      mask Help: eval('blocksethelp');
      mask TypeOptions trig: Rising edge | Falling edge | Either edge
      mask Display: disp('S/H')
  Sample and Hold1 : dspsigops/Sample and Hold  SystemSampleTime=-1  trig=Rising edge  initCond=0  latchinput=off
  Sample and Hold2 : Subsystem  TreatAsAtomicUnit=on  mask(Sample and Hold){trig=Rising edge, initCond=0, latchinput=off}
      mask prompts: trig "Trigger type:"; initCond "Initial condition:"; latchinput "Latch (buffer) input"
      mask help: Sample and hold the input signal. If Latch (buffer) input is selected, then this block produces the value of the input from the previous time step.
      mask init: same as WaveletTraj/Wavelet Trajectory/TrajGen1/Input Latching/Sample and Hold2
      mask Help: eval('blocksethelp');
      mask TypeOptions trig: Rising edge | Falling edge | Either edge
      mask Display: disp('S/H')
  Sample and Hold3 : dspsigops/Sample and Hold  SystemSampleTime=-1  trig=Rising edge  initCond=0  latchinput=off
  Sample and Hold4 : Subsystem  TreatAsAtomicUnit=on  mask(Sample and Hold){trig=Rising edge, initCond=0, latchinput=off}
      mask prompts: trig "Trigger type:"; initCond "Initial condition:"; latchinput "Latch (buffer) input"
      mask help: Sample and hold the input signal. If Latch (buffer) input is selected, then this block produces the value of the input from the previous time step.
      mask init: same as WaveletTraj/Wavelet Trajectory/TrajGen1/Input Latching/Sample and Hold
      mask Help: eval('blocksethelp');
      mask TypeOptions trig: Rising edge | Falling edge | Either edge
      mask Display: disp('S/H')
  Sample and Hold5 : Subsystem  TreatAsAtomicUnit=on  mask(Sample and Hold){trig=Rising edge, initCond=0, latchinput=off}
      mask prompts: trig "Trigger type:"; initCond "Initial condition:"; latchinput "Latch (buffer) input"
      mask help: Sample and hold the input signal. If Latch (buffer) input is selected, then this block produces the value of the input from the previous time step.
      mask init: same as WaveletTraj/Wavelet Trajectory/TrajGen1/Input Latching/Sample and Hold5
      mask Help: eval('blocksethelp');
      mask TypeOptions trig: Rising edge | Falling edge | Either edge
      mask Display: disp('S/H')
  Sample and Hold6 : dspsigops/Sample and Hold  SystemSampleTime=-1  trig=Rising edge  initCond=0  latchinput=off
  Saturation : Saturate  UpperLimit=2  LowerLimit=0  OutDataTypeStr=uint8  RndMeth=Nearest
  trigger_trg : Outport
  abort_trg : Outport  Port=2
  mode_lt : Outport  Port=3
  int_mode_lt : Outport  Port=4
  Res_lt : Outport  Port=5
  N_lt : Outport  Port=6
  x0_lt : Outport  Port=7
  mul_lt : Outport  Port=8
  T1 : Outport  Port=9
  c_lt : Outport  Port=10
  wires:
  Saturation/1 -> Sample and Hold3/1, Sample and Hold/1(mode), Sample and Hold5/1(mode), Sample and Hold4/1(mode)
  int_mode/1 -> Sample and Hold6/1
  Sample and Hold6/1 -> int_mode_lt/1
  Sample and Hold3/1 -> mode_lt/1
  Edge Detector1/1 -> abort_trg/1
  abort/1 -> Edge Detector1/1
  c/1 -> Sample and Hold4/2(In)
  Sample and Hold5/1(" ") -> mul_lt/1
  xf/1 -> Sample and Hold5/3(xf)
  mode/1 -> Saturation/1
  trigger/1 -> Sample and Hold6/Trigger, Sample and Hold/Trigger, Sample and Hold4/Trigger, Sample and Hold2/Trigger, Sample and Hold5/Trigger, Sample and Hold1/Trigger, Sample and Hold3/Trigger, Edge Detector/1
  Edge Detector/1 -> trigger_trg/1
  Sample and Hold/1(" ") -> Res_lt/1
  Res/1 -> Sample and Hold/2(In)
  Sample and Hold/2(" 1") -> N_lt/1
  x0/1 -> Sample and Hold5/2(x0), Sample and Hold1/1
  Sample and Hold1/1 -> x0_lt/1
  T/1 -> Sample and Hold2/1(In)
  Sample and Hold2/1(" ") -> T1/1
  Sample and Hold4/1(" ") -> c_lt/1

== system WaveletTraj/Wavelet Trajectory/TrajGen1/Compute Join Coeffs/Derivative1 in tau ==
  Res : Inport
  tau : Inport  Port=2
  c : Inport  Port=3
  N : Inport  Port=4
  Derivative : Subsystem  RTWFcnName=Trajectory_Derivative
  out : Outport
  wires:
  N/1 -> Derivative/4(N)
  c/1 -> Derivative/3(c)
  Derivative/1(Dout) -> out/1
  tau/1 -> Derivative/2(tau)
  Res/1 -> Derivative/1(Res)

== system WaveletTraj/Wavelet Trajectory/TrajGen1/Compute Join Coeffs/Derivative2 in 0 ==
  Res : Inport
  tau : Inport  Port=2
  c : Inport  Port=3
  N : Inport  Port=4
  Derivative : Subsystem  RTWFcnName=Trajectory_Derivative
  out : Outport
  wires:
  Res/1 -> Derivative/1(Res)
  tau/1 -> Derivative/2(tau)
  Derivative/1(Dout) -> out/1
  c/1 -> Derivative/3(c)
  N/1 -> Derivative/4(N)

== system WaveletTraj/Wavelet Trajectory/TrajGen1/Compute Join Coeffs/Derivative2 in tau1 ==
  Res : Inport
  tau : Inport  Port=2
  c : Inport  Port=3
  N : Inport  Port=4
  Derivative : Subsystem  RTWFcnName=Trajectory_Derivative
  out : Outport
  wires:
  N/1 -> Derivative/4(N)
  c/1 -> Derivative/3(c)
  Derivative/1(Dout) -> out/1
  tau/1 -> Derivative/2(tau)
  Res/1 -> Derivative/1(Res)

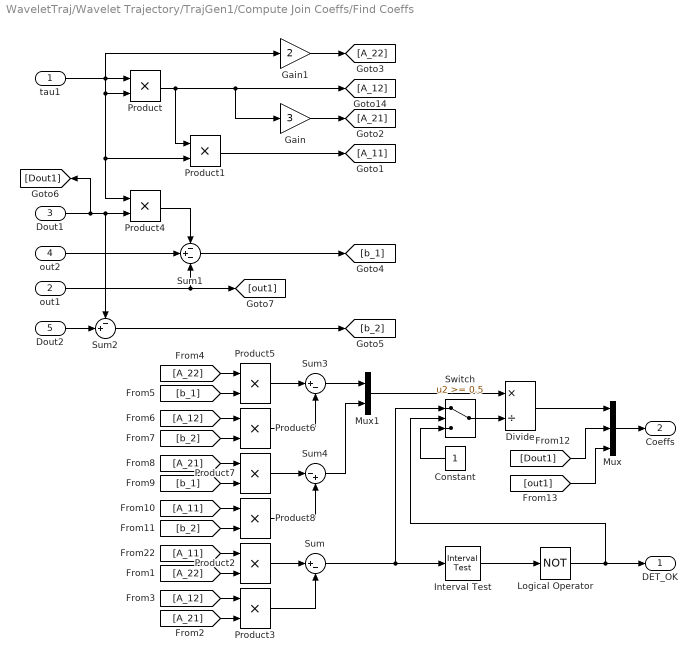
== system WaveletTraj/Wavelet Trajectory/TrajGen1/Compute Join Coeffs/Find Coeffs ==
  tau1 : Inport
  out1 : Inport  Port=2
  Dout1 : Inport  Port=3
  out2 : Inport  Port=4
  Dout2 : Inport  Port=5
  Constant : Constant  OutDataTypeStr=fixdt(1,w,f)
  Divide : Product  Inputs=*/  OutDataTypeStr=fixdt(1,w,f)  RndMeth=Nearest  SaturateOnIntegerOverflow=on
  Gain : Gain  Gain=3  RndMeth=Nearest  SaturateOnIntegerOverflow=on  OutDataTypeStr=Inherit: Same as input  ParamDataTypeStr=Inherit: Same as input
  Gain1 : Gain  Gain=2  RndMeth=Nearest  SaturateOnIntegerOverflow=on  OutDataTypeStr=Inherit: Same as input  ParamDataTypeStr=Inherit: Same as input
  Interval Test : simulink/Logic and Bit Operations/Interval Test  SystemSampleTime=-1  IntervalClosedRight=on  uplimit=2^-f  IntervalClosedLeft=on  lowlimit=-2^-f  LogicOutDataTypeMode=boolean
  Logical Operator : Logic  Operator=NOT  IconShape=distinctive  AllPortsSameDT=off  OutDataTypeStr=boolean
  Mux : Mux  Inputs=3
  Mux1 : Mux  Inputs=2
  Product{,1..8} (9 alike) : Product  OutDataTypeStr=fixdt(1,w,f)  RndMeth=Nearest  SaturateOnIntegerOverflow=on
  Sum : Sum  Inputs=|+-  OutDataTypeStr=fixdt(1,w,f)  RndMeth=Nearest  SaturateOnIntegerOverflow=on
  Sum1 : Sum  Inputs=-+-  OutDataTypeStr=fixdt(1,w,f)  RndMeth=Nearest  SaturateOnIntegerOverflow=on
  Sum2 : Sum  Inputs=-+|  OutDataTypeStr=fixdt(1,w,f)  RndMeth=Nearest  SaturateOnIntegerOverflow=on
  Sum3 : Sum  Inputs=|+-  OutDataTypeStr=fixdt(1,w,f)  RndMeth=Nearest  SaturateOnIntegerOverflow=on
  Sum4 : Sum  Inputs=|-+  OutDataTypeStr=fixdt(1,w,f)  RndMeth=Nearest  SaturateOnIntegerOverflow=on
  Switch : Switch  Threshold=0.5  OutDataTypeStr=fixdt(1,w,f)  RndMeth=Nearest  SaturateOnIntegerOverflow=on
  DET_OK : Outport
  Coeffs : Outport  Port=2
  wires:
  Constant/1 -> Switch/3
  Switch/1 -> Divide/2
  Logical Operator/1 -> Switch/2, DET_OK/1
  Interval Test/1 -> Logical Operator/1
  Mux/1 -> Coeffs/1
  [out1] -> Mux/3
  [Dout1] -> Mux/2
  Divide/1 -> Mux/1
  Sum/1 -> Switch/1, Interval Test/1
  Mux1/1 -> Divide/1
  Sum4/1 -> Mux1/2
  Sum3/1 -> Mux1/1
  Product8/1 -> Sum4/2
  Product7/1 -> Sum4/1
  [b_2] -> Product8/2
  [A_11] -> Product8/1
  [b_1] -> Product7/2
  [A_21] -> Product7/1
  Product6/1 -> Sum3/2
  Product5/1 -> Sum3/1
  [b_2] -> Product6/2
  [A_12] -> Product6/1
  [b_1] -> Product5/2
  [A_22] -> Product5/1
  Sum2/1 -> [b_2]
  Sum1/1 -> [b_1]
  Dout2/1 -> Sum2/2
  Product4/1 -> Sum1/1
  out1/1 -> [out1], Sum1/3
  out2/1 -> Sum1/2
  Dout1/1 -> [Dout1], Sum2/1, Product4/2
  Product3/1 -> Sum/2
  Product2/1 -> Sum/1
  [A_21] -> Product3/2
  [A_12] -> Product3/1
  [A_22] -> Product2/2
  [A_11] -> Product2/1
  Gain1/1 -> [A_22]
  Gain/1 -> [A_21]
  Product1/1 -> [A_11]
  Product/1 -> Gain/1, [A_12], Product1/1
  tau1/1 -> Gain1/1, Product4/1, Product1/2, Product/2, Product/1

== system WaveletTraj/Wavelet Trajectory/TrajGen1/Compute Join Coeffs/Position2 in tau1 ==
  Res : Inport
  tau : Inport  Port=2
  c : Inport  Port=3
  N : Inport  Port=4
  Position : Subsystem  RTWFcnName=Trajectory_Position
  out : Outport
  wires:
  Res/1 -> Position/1(Res)
  tau/1 -> Position/2(tau)
  Position/1(out) -> out/1
  c/1 -> Position/3(c)
  N/1 -> Position/4(N)

== system WaveletTraj/Wavelet Trajectory/TrajGen1/Compute Join Output/CalcPoly ==
  tau : Inport
  Coeffs : Inport  Port=2
  Add : Sum  Inputs=4  OutDataTypeStr=fixdt(1,w,f)  RndMeth=Nearest  SaturateOnIntegerOverflow=on
  Demux : Demux
  Product{,1..4} (5 alike) : Product  OutDataTypeStr=fixdt(1,w,f)  RndMeth=Nearest  SaturateOnIntegerOverflow=on
  out_poly3 : Outport
  wires:
  Coeffs/1 -> Demux/1
  Add/1 -> out_poly3/1
  Demux/4 -> Add/4
  Product4/1 -> Add/3
  Product2/1 -> Add/2
  Product3/1 -> Add/1
  Demux/3 -> Product4/2
  Demux/2 -> Product3/2
  Demux/1 -> Product2/2
  Product1/1 -> Product2/1
  Product/1 -> Product3/1, Product1/1
  tau/1 -> Product4/1, Product1/2, Product/2, Product/1
